simulink model "lab_2_3"  (R2024a)
settings: Solver=VariableStepAuto  StartTime=0.0  StopTime=25  RelTol=1e-3
settings Model: Creator=lw53894  LastModifiedBy=lw53894

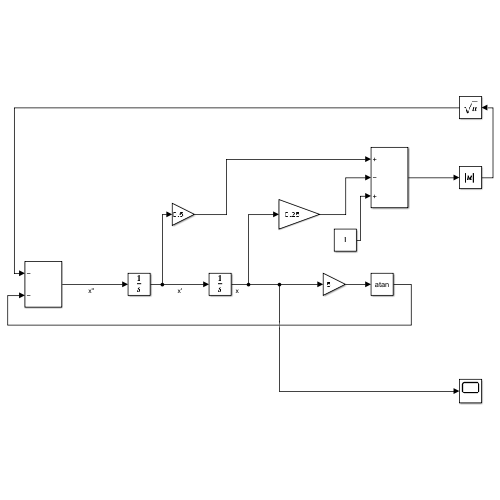
[thumbnail: Simulink's stored preview of the top-level diagram]
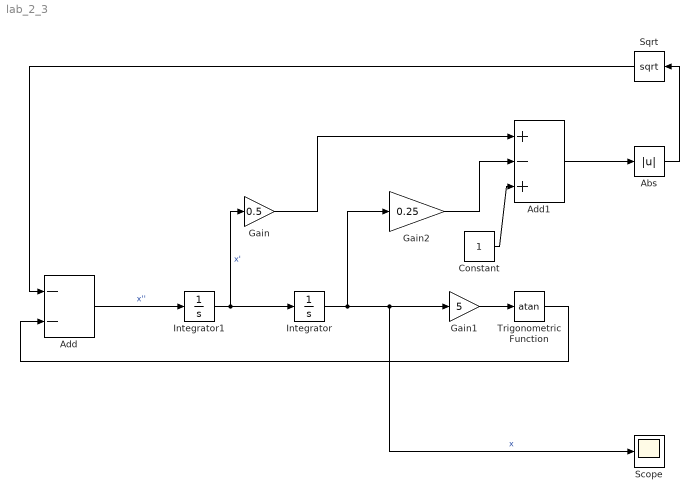
== system lab_2_3 ==
  Abs : Abs  SaturateOnIntegerOverflow=off
  Add : Sum  Inputs=--
  Add1 : Sum  Inputs=+-+
  Constant : Constant
  Gain : Gain  Gain=0.5
  Gain1 : Gain  Gain=5
  Gain2 : Gain  Gain=0.25
  Integrator : Integrator  InitialCondition=1
  Integrator1 : Integrator
  Scope : Scope
  Sqrt : Sqrt
  Trigonometric Function : Trigonometry  Operator=atan
  wires:
  Integrator1/1 -> Gain/1, Integrator/1  "x'"
  Add/1 -> Integrator1/1  "x''"
  Integrator/1 -> Gain2/1, Scope/1, Gain1/1  "x"
  Gain1/1 -> Trigonometric Function/1
  Gain/1 -> Add1/1
  Gain2/1 -> Add1/2
  Constant/1 -> Add1/3
  Add1/1 -> Abs/1
  Trigonometric Function/1 -> Add/2
  Abs/1 -> Sqrt/1
  Sqrt/1 -> Add/1
